simulink model "LiniowyTransmitancje"  (R2015a)
settings: Solver=ode45  StartTime=0.0  StopTime=200  MaxStep=0.1  RelTol=1e-3
values from neighbouring files (symbols this model uses):
  a1 = Aw1*sqrt(2*g)    [Dodatkowe.m]    (also in Dodatkowe2.m; ZbiorniczkiLiniowe.m; ZbiorniczkiSumaryczne.m)
  A1 = 3500    [Dodatkowe.m]    (also in Dodatkowe2.m; ZbiorniczkiLiniowe.m; ZbiorniczkiSumaryczne.m)
  A2 = 2000    [Dodatkowe.m]    (also in Dodatkowe2.m; ZbiorniczkiLiniowe.m; ZbiorniczkiSumaryczne.m)
  a2 = Aw2*sqrt(2*g)    [Dodatkowe.m]    (also in Dodatkowe2.m; ZbiorniczkiLiniowe.m; ZbiorniczkiSumaryczne.m)
  df1 = 200    [Dodatkowe.m]    (also in Dodatkowe2.m; ZbiorniczkiLiniowe.m; ZbiorniczkiSumaryczne.m)
  df2 = 0    [Dodatkowe.m]    (also in Dodatkowe2.m; ZbiorniczkiLiniowe.m; ZbiorniczkiSumaryczne.m)
  h1 = ((f1.^2)/((Aw1.^2)*2*g))+((f1+f2).^2)/((Aw2.^2)*2*g)    [Dodatkowe.m]    (also in Dodatkowe2.m; ZbiorniczkiLiniowe.m = (f1/a1)+(f1+df2)/a2; ZbiorniczkiSumaryczne.m = (f1/a1)+(f1+df2)/a2)
  h2 = ((f1+f2).^2)/((Aw2.^2)*2*g)    [Dodatkowe.m]    (also in Dodatkowe2.m; ZbiorniczkiLiniowe.m = (f1+df2)/a2; ZbiorniczkiSumaryczne.m = (f1+df2)/a2)
  t1 = 40    [Dodatkowe.m]    (also in Dodatkowe2.m; ZbiorniczkiLiniowe.m; ZbiorniczkiSumaryczne.m)
  t2 = 40    [Dodatkowe.m]    (also in Dodatkowe2.m; ZbiorniczkiLiniowe.m; ZbiorniczkiSumaryczne.m)
settings Model: Creator=apuch  LastModifiedBy=apuch

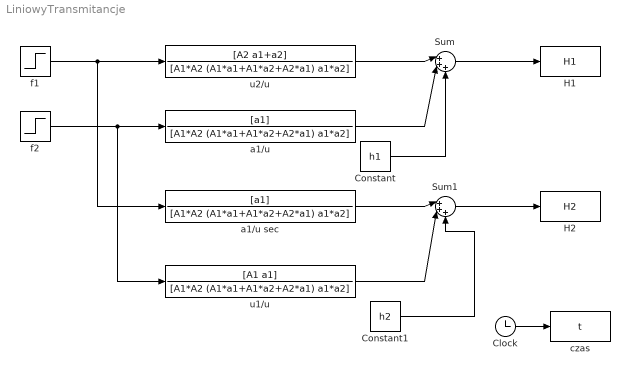
== system LiniowyTransmitancje ==
  Clock : Clock
  Constant : Constant  Value=h1
  Constant1 : Constant  Value=h2
  H1 : ToWorkspace  VariableName=H1  SampleTime=-1
  H2 : ToWorkspace  VariableName=H2  SampleTime=-1
  Sum : Sum  Inputs=|+++
  Sum1 : Sum  Inputs=|+++
  a1/u : TransferFcn  Numerator=[a1]  Denominator=[A1*A2 (A1*a1+A1*a2+A2*a1) a1*a2]
  a1/u sec : TransferFcn  Numerator=[a1]  Denominator=[A1*A2 (A1*a1+A1*a2+A2*a1) a1*a2]
  czas : ToWorkspace  VariableName=t  SampleTime=-1
  f1 : Step  Time=t1  After=df1  SampleTime=0
  "f2 " : Step  Time=t2  After=df2  SampleTime=0
  u1/u : TransferFcn  Numerator=[A1 a1]  Denominator=[A1*A2 (A1*a1+A1*a2+A2*a1) a1*a2]
  u2/u : TransferFcn  Numerator=[A2 a1+a2]  Denominator=[A1*A2 (A1*a1+A1*a2+A2*a1) a1*a2]
  wires:
  f1/1 -> a1/u sec/1, u2/u/1
  "f2 "/1 -> u1/u/1, a1/u/1
  u2/u/1 -> Sum/1
  a1/u/1 -> Sum/2
  Sum/1 -> H1/1
  a1/u sec/1 -> Sum1/1
  u1/u/1 -> Sum1/2
  Sum1/1 -> H2/1
  Clock/1 -> czas/1
  Constant1/1 -> Sum1/3
  Constant/1 -> Sum/3
